simulink model "sin_power"  (Simulink 7.3)
settings: Solver=VariableStepDiscrete  StartTime=0.0  StopTime=0.2  RelTol=1e-3
libraries: powerlib x5
settings Model: Creator=sn00632  LastModifiedBy=sn00632

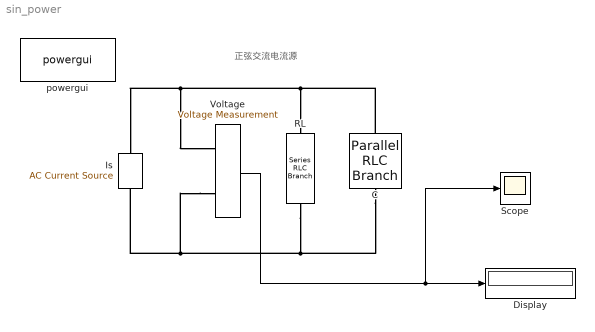
== system sin_power ==
  note: 正弦交流电流源
  C : powerlib/Elements/Parallel RLC Branch  DialogController=POWERSYS.PowerSysDialog  PhysicalDomain=powersysdomain  SubClassName=unknown  LeftPortType=p1  RightPortType=p1  LConnTagsString=a  RConnTagsString=__new0  BranchType=C  Resistance=1  Inductance=1e-3  SetiL0=off  InitialCurrent=0  Capacitance=5e-4  Setx0=off  InitialVoltage=0  Measurements=None
  Display : Display
  Is : powerlib/Electrical Sources/AC Current Source  DialogController=POWERSYS.PowerSysDialog  SystemSampleTime=-1  Amplitude=10*sqrt(2)  Phase=15  Frequency=100  SampleTime=0  Measurements=None
  RL : powerlib/Elements/Series RLC Branch  DialogController=POWERSYS.PowerSysDialog  PhysicalDomain=powersysdomain  SubClassName=unknown  LeftPortType=p1  RightPortType=p1  LConnTagsString=__new0  RConnTagsString=__new0  BranchType=RL  Resistance=10  Inductance=0.1  SetiL0=off  InitialCurrent=0  Capacitance=1.0  Setx0=off  InitialVoltage=0  Measurements=None
  Scope : Scope
      settings: YMin=-50  YMax=50
  Voltage : powerlib/Measurements/Voltage Measurement  DialogController=POWERSYS.PowerSysDialog  SystemSampleTime=-1  PhasorSimulation=off  OutputType=Complex  PSBequivalent=0
  powergui : powerlib/powergui  Priority=1  SystemSampleTime=-1  SimulationMode=Discrete  SampleTime=50e-6  frequency=60  SPID=off  DisableSnubberDevices=off  DisableRonSwitches=off  DisableVfSwitches=off  SwTol=0  Interpol=off  frequencyindice=100  echomessages=off  HookPort=off  DisplayEquations=off  FunctionMessages=off  EnableUseOfTLC=off  x0status=blocks  RestoreLinks=warning  Frange=[0:2:500]  Ylog=off  Xlog=on  ShowGrid=off  save=off  variable=ZData  ZoomFFT=on  StartTime=0.0  cycles=1  DisplayStyle=1  fundamental=60  FreqAxis=off  MaxFrequency=1000  frequencyindicesteady=1  RmsSteady=1  display=off  Ts=0  methode=off
  wires:
  Voltage/1 -> Display/1, Scope/1
  connections:
  C/LConn1 -- RL/LConn1 -- Is/RConn1 -- Voltage/LConn1
  Voltage/LConn2 -- C/RConn1 -- RL/RConn1 -- Is/LConn1
